simulink model "MAS23_sim"  (R2018b)
settings: Solver=VariableStepAuto  StartTime=0.0  StopTime=tps_sim  MaxStep=1e-4  RelTol=1e-3
values from neighbouring files (symbols this model uses):
  alpha = 4e-3    (= 0.004)    [MAS23_init.m]
  C_in = Cn    (= 643)    [MAS23_init.m]
  Cemn = Cn + pm/Wn    (= 647.177013984)    [MAS23_init.m]
  Concordia = sqrt(2/3)*[1 -0.5 -0.5;0 sqrt(3)/2 -sqrt(3)/2;1/sqrt(2) 1/sqrt(2) 1/sqrt(2)]    [MAS23_init.m]
  decider_R = 1    [MAS23_init.m]
  deciderC = 1    [MAS23_init.m]
  deciderC2 = 1    [MAS23_init.m]
  echauffement = 200    [MAS23_init.m]
  f = u(3)*u(2)/u(1)    [FluxCloche.m]    (also in MAS23_init.m = 0.0131717538735)
  Frdn_max = Frdn*sqrt(2)    [MAS23_init.m]
  IConcordia = inv(Concordia)    [MAS23_init.m]
  IFlux = inv(Flux)    [MAS23_init.m]
  J = 1.92    [MAS23_init.m]
  kc = Cn/Wn    (= 2.06601537836)    [MAS23_init.m]
  Kc = 1.6*3*to_c/sigma/Ts/(P*Msr^2/Lr*Imr_refn/Rs)    [MAS23_init.m]
  Kf = 0.02*3/Tr    [MAS23_init.m]
  Kv = 3    [MAS23_init.m]
  Lr = Lrr-Mr    [MAS23_init.m]
  Ls = Lss-Ms    [MAS23_init.m]
  Msr = 3/2*Msri    [MAS23_init.m]
  N_in = Nn    (= 2972)    [MAS23_init.m]
  P = 1    [MAS23_init.m]
  Rr = Rs    [MAS23_init.m]
  Rs = Rp2    [MAS23_init.m]
  sigma = 1-Msr^2/Ls/Lr    [MAS23_init.m]
  tau = 2    [MAS23_init.m]
  to_c = 0.0055    [MAS23_init.m]
  to_f = 1/(-poleF(2))    [MAS23_init.m]
  to_v = J/k    (= 145.766465001)    [MAS23_init.m]
  Tr = Lr/Rr    [MAS23_init.m]
  Wb = 2*pi*freq    (= 314.159265359)    [MAS23_init.m]
settings Model: Creator=Louis  LastModifiedBy=Louis
settings DataIOCC: SaveOutput=off  SignalLogging=off  DSMLogging=off  SaveTime=off  TimeSaveName=T

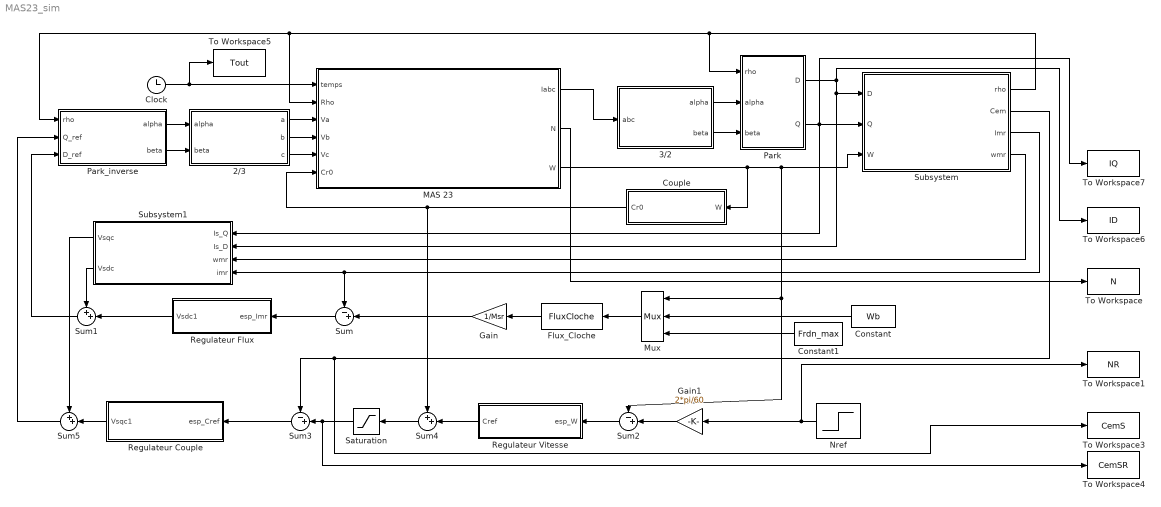
== system MAS23_sim ==
  2/3 : Subsystem
  3/2 : Subsystem
  Clock : Clock
  Constant : Constant  Value=Wb
  Constant1 : Constant  Value=Frdn_max
  Couple : Subsystem
  Flux_Cloche : MATLABFcn  MATLABFcn=FluxCloche  OutputDimensions=1
  Gain : Gain  Gain=1/Msr
  Gain1 : Gain  Gain=2*pi/60
  MAS 23 : Subsystem
      mask Display: image(imread('electricmotor.jpg'));
  Mux : Mux  Inputs=3
  Nref : Step  Time=2  After=N_in  SampleTime=0
  Park : Subsystem
  Park_inverse : Subsystem
  Regulateur Couple : Subsystem
  Regulateur Flux : Subsystem
  Regulateur Vitesse : Subsystem
  Saturation : Saturate  UpperLimit=Cemn  LowerLimit=-Cemn
  Subsystem : Subsystem
  Subsystem1 : Subsystem
  Sum : Sum  Inputs=-+|
  Sum1 : Sum  Inputs=++|
  Sum2 : Sum  Inputs=-+|
  Sum3 : Sum  Inputs=-+|
  Sum4 : Sum  Inputs=++|
  Sum5 : Sum  Inputs=++|
  To Workspace : ToWorkspace  VariableName=N  SampleTime=-1
  To Workspace1 : ToWorkspace  VariableName=NR  SampleTime=-1
  To Workspace3 : ToWorkspace  VariableName=CemS  SampleTime=-1
  To Workspace4 : ToWorkspace  VariableName=CemSR  SampleTime=-1
  To Workspace5 : ToWorkspace  VariableName=Tout  SampleTime=-1
  To Workspace6 : ToWorkspace  VariableName=ID  SampleTime=-1
  To Workspace7 : ToWorkspace  VariableName=IQ  SampleTime=-1
  wires:
  MAS 23/1(Iabc) -> 3/2/1(abc)
  3/2/1(alpha) -> Park/2(alpha)
  3/2/2(beta) -> Park/3(beta)
  Park_inverse/1(alpha) -> 2/3/1(alpha)
  Park_inverse/2(beta) -> 2/3/2(beta)
  2/3/1(a) -> MAS 23/3(Va)
  2/3/2(b) -> MAS 23/4(Vb)
  2/3/3(c) -> MAS 23/5(Vc)
  Subsystem/1(rho) -> Park/1(rho), MAS 23/2(Rho), Park_inverse/1(rho)
  Park/2(Q) -> Subsystem/2(Q), Subsystem1/1(Is_Q), To Workspace7/1
  MAS 23/3(W) -> Couple/1(W), Sum2/1, Mux/1, Subsystem/3(W)
  Park/1(D) -> Subsystem1/2(Is_D), Subsystem/1(D), To Workspace6/1
  Subsystem/4(wmr) -> Subsystem1/3(wmr)
  Subsystem/3(Imr) -> Sum/1, Subsystem1/4(imr)
  Constant/1 -> Mux/2
  Constant1/1 -> Mux/3
  Mux/1 -> Flux_Cloche/1
  Flux_Cloche/1 -> Gain/1
  Gain/1 -> Sum/2
  Sum/1 -> Regulateur Flux/1(esp_Imr)
  Regulateur Flux/1(Vsdc1) -> Sum1/2
  Subsystem1/2(Vsdc) -> Sum1/1
  Sum1/1 -> Park_inverse/3(D_ref)
  Nref/1 -> To Workspace1/1, Gain1/1
  Gain1/1 -> Sum2/2
  Sum2/1 -> Regulateur Vitesse/1(esp_W)
  Subsystem/2(Cem) -> To Workspace3/1, Sum3/1
  Sum3/1 -> Regulateur Couple/1(esp_Cref)
  Regulateur Vitesse/1(Cref) -> Sum4/2
  Saturation/1 -> To Workspace4/1, Sum3/2
  Subsystem1/1(Vsqc) -> Sum5/1
  Sum5/1 -> Park_inverse/2(Q_ref)
  MAS 23/2(N) -> To Workspace/1
  Couple/1(Cr0) -> Sum4/1, MAS 23/6(Cr0)
  Regulateur Couple/1(Vsqc1) -> Sum5/2
  Sum4/1 -> Saturation/1
  Clock/1 -> To Workspace5/1, MAS 23/1(temps)

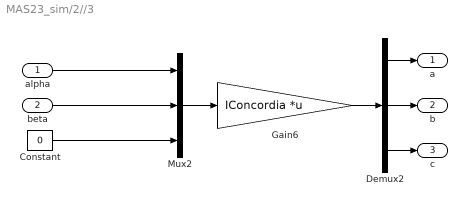
== system MAS23_sim/2//3 ==
  alpha : Inport
  beta : Inport  Port=2
  Constant : Constant  Value=0
  Demux2 : Demux  Outputs=3
  Gain6 : Gain  Gain=IConcordia  Multiplication=Matrix(K*u) (u vector)
  Mux2 : Mux  Inputs=3
  a : Outport
  b : Outport  Port=2
  c : Outport  Port=3
  wires:
  Demux2/1 -> a/1
  Demux2/2 -> b/1
  alpha/1 -> Mux2/1
  Constant/1 -> Mux2/3
  beta/1 -> Mux2/2
  Gain6/1 -> Demux2/1
  Demux2/3 -> c/1
  Mux2/1 -> Gain6/1

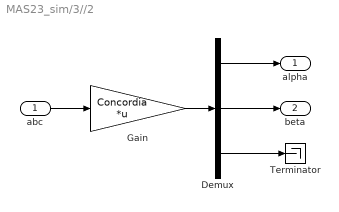
== system MAS23_sim/3//2 ==
  abc : Inport
  Demux : Demux  Outputs=3
  Gain : Gain  Gain=Concordia  Multiplication=Matrix(K*u) (u vector)
  Terminator : Terminator
  alpha : Outport
  beta : Outport  Port=2
  wires:
  Gain/1 -> Demux/1
  Demux/3 -> Terminator/1
  Demux/2 -> beta/1
  abc/1 -> Gain/1
  Demux/1 -> alpha/1

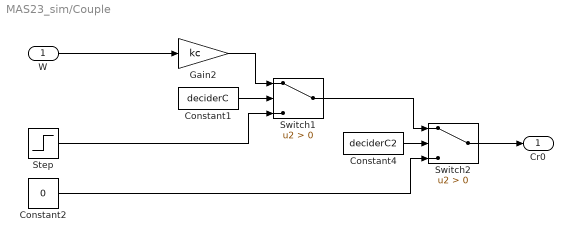
== system MAS23_sim/Couple ==
  W : Inport
  Constant1 : Constant  Value=deciderC
  Constant2 : Constant  Value=0
  Constant4 : Constant  Value=deciderC2
  Gain2 : Gain  Gain=kc
  Step : Step  Time=6  After=C_in  SampleTime=0
  Switch1 : Switch  Criteria=u2 > Threshold
  Switch2 : Switch  Criteria=u2 > Threshold
  Cr0 : Outport
  wires:
  W/1 -> Gain2/1
  Gain2/1 -> Switch1/1
  Constant1/1 -> Switch1/2
  Step/1 -> Switch1/3
  Switch1/1 -> Switch2/1
  Constant2/1 -> Switch2/3
  Constant4/1 -> Switch2/2
  Switch2/1 -> Cr0/1

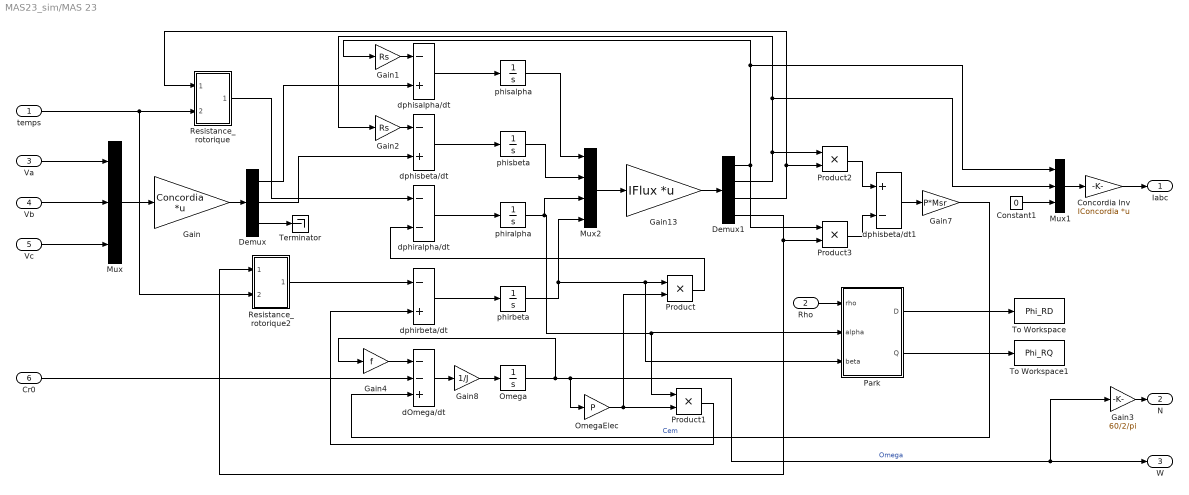
== system MAS23_sim/MAS 23 ==
  temps : Inport
  Rho : Inport  Port=2
  Va : Inport  Port=3
  Vb : Inport  Port=4
  Vc : Inport  Port=5
  Cr0 : Inport  Port=6
  Concordia Inv : Gain  Gain=IConcordia  Multiplication=Matrix(K*u) (u vector)
  Constant1 : Constant  Value=0
  Demux : Demux  Outputs=3
  Demux1 : Demux
  Gain : Gain  Gain=Concordia  Multiplication=Matrix(K*u) (u vector)
  Gain1 : Gain  Gain=Rs
  Gain13 : Gain  Gain=IFlux  Multiplication=Matrix(K*u) (u vector)
  Gain2 : Gain  Gain=Rs
  Gain3 : Gain  Gain=60/2/pi
  Gain4 : Gain  Gain=f
  Gain7 : Gain  Gain=P*Msr
  Gain8 : Gain  Gain=1/J
  Mux : Mux  Inputs=3
  Mux1 : Mux  Inputs=3
  Mux2 : Mux
  Omega : Integrator
  OmegaElec : Gain  Gain=P
  Park : Subsystem
  Product{,1..3} (4 alike) : Product
  Resistance_rotorique : Subsystem
  Resistance_rotorique2 : Subsystem
  Terminator : Terminator
  To Workspace : ToWorkspace  VariableName=Phi_RD  SampleTime=-1
  To Workspace1 : ToWorkspace  VariableName=Phi_RQ  SampleTime=-1
  dOmega/dt : Sum  Inputs=--+
  dphiralpha/dt : Sum  Inputs=--
  dphirbeta/dt : Sum  Inputs=-+
  dphisalpha/dt : Sum  Inputs=-+
  dphisbeta/dt : Sum  Inputs=-+
  dphisbeta/dt1 : Sum  Inputs=+-
  phiralpha : Integrator
  phirbeta : Integrator
  phisalpha : Integrator
  phisbeta : Integrator
  Iabc : Outport
  N : Outport  Port=2
  W : Outport  Port=3
  wires:
  Vc/1 -> Mux/3
  phisalpha/1 -> Mux2/1
  Mux2/1 -> Gain13/1
  Va/1 -> Mux/1
  phirbeta/1 -> Mux2/4, Product/1, Park/3(beta)
  dphisalpha/dt/1 -> phisalpha/1
  Gain13/1 -> Demux1/1
  dphirbeta/dt/1 -> phirbeta/1
  Product/1 -> dphiralpha/dt/2
  Demux/2 -> dphisbeta/dt/2
  Gain/1 -> Demux/1
  Product1/1 -> dphirbeta/dt/2
  phisbeta/1 -> Mux2/2
  Gain7/1 -> dOmega/dt/3  "Cem"
  dphisbeta/dt1/1 -> Gain7/1
  Mux1/1 -> Concordia Inv/1
  Product3/1 -> dphisbeta/dt1/2
  Gain1/1 -> dphisalpha/dt/1
  phiralpha/1 -> Product1/1, Park/2(alpha), Mux2/3
  Demux/3 -> Terminator/1
  Gain2/1 -> dphisbeta/dt/1
  dphisbeta/dt/1 -> phisbeta/1
  Demux/1 -> dphisalpha/dt/2
  Gain8/1 -> Omega/1
  Gain4/1 -> dOmega/dt/1
  Demux1/1 -> Gain1/1, Mux1/1, Product3/1
  Mux/1 -> Gain/1
  Product2/1 -> dphisbeta/dt1/1
  Constant1/1 -> Mux1/3
  Demux1/4 -> Resistance_rotorique2/1(In1), Product3/2
  OmegaElec/1 -> Product1/2, Product/2
  dphiralpha/dt/1 -> phiralpha/1
  Vb/1 -> Mux/2
  Demux1/2 -> Gain2/1, Mux1/2, Product2/1
  dOmega/dt/1 -> Gain8/1
  Omega/1 -> Gain4/1, Gain3/1, W/1, OmegaElec/1  "Omega"
  Demux1/3 -> Resistance_rotorique/1(In1), Product2/2
  Resistance_rotorique2/1(Out1) -> dphirbeta/dt/1
  Resistance_rotorique/1(Out1) -> dphiralpha/dt/1
  Cr0/1 -> dOmega/dt/2
  Concordia Inv/1 -> Iabc/1
  Rho/1 -> Park/1(rho)
  Park/1(D) -> To Workspace/1
  Park/2(Q) -> To Workspace1/1
  temps/1 -> Resistance_rotorique2/2(Time), Resistance_rotorique/2(Time)
  Gain3/1 -> N/1

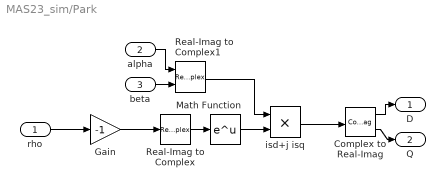
== system MAS23_sim/Park ==
  rho : Inport
  alpha : Inport  Port=2
  beta : Inport  Port=3
  Complex to Real-Imag : ComplexToRealImag
  Gain : Gain  Gain=-1
  Math Function : Math  SaturateOnIntegerOverflow=on
  Real-Imag to Complex : RealImagToComplex  Input=Imag
  Real-Imag to Complex1 : RealImagToComplex
  isd+j isq : Product
  D : Outport
  Q : Outport  Port=2
  wires:
  Complex to Real-Imag/1 -> D/1
  Complex to Real-Imag/2 -> Q/1
  rho/1 -> Gain/1
  alpha/1 -> Real-Imag to Complex1/1
  beta/1 -> Real-Imag to Complex1/2
  Real-Imag to Complex/1 -> Math Function/1
  Real-Imag to Complex1/1 -> isd+j isq/1
  Gain/1 -> Real-Imag to Complex/1
  isd+j isq/1 -> Complex to Real-Imag/1
  Math Function/1 -> isd+j isq/2

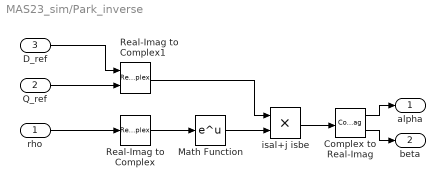
== system MAS23_sim/Park_inverse ==
  rho : Inport
  Q_ref : Inport  Port=2
  D_ref : Inport  Port=3
  Complex to Real-Imag : ComplexToRealImag
  Math Function : Math  SaturateOnIntegerOverflow=on
  Real-Imag to Complex : RealImagToComplex  Input=Imag
  Real-Imag to Complex1 : RealImagToComplex
  isal+j isbe : Product
  alpha : Outport
  beta : Outport  Port=2
  wires:
  Q_ref/1 -> Real-Imag to Complex1/2
  D_ref/1 -> Real-Imag to Complex1/1
  Math Function/1 -> isal+j isbe/2
  isal+j isbe/1 -> Complex to Real-Imag/1
  rho/1 -> Real-Imag to Complex/1
  Real-Imag to Complex1/1 -> isal+j isbe/1
  Real-Imag to Complex/1 -> Math Function/1
  Complex to Real-Imag/2 -> beta/1
  Complex to Real-Imag/1 -> alpha/1

== system MAS23_sim/Regulateur Couple ==
  esp_Cref : Inport
  Cc : TransferFcn  Numerator=[to_c 1]  Denominator=[to_c 0]
  Gain3 : Gain  Gain=Kc
  Vsqc1 : Outport
  wires:
  Gain3/1 -> Cc/1
  esp_Cref/1 -> Gain3/1
  Cc/1 -> Vsqc1/1

== system MAS23_sim/Regulateur Flux ==
  esp_Imr : Inport
  Cp : TransferFcn  Numerator=[to_f 1]  Denominator=[to_f 0]
  Gain1 : Gain  Gain=Kf
  Vsdc1 : Outport
  wires:
  Gain1/1 -> Cp/1
  Cp/1 -> Vsdc1/1
  esp_Imr/1 -> Gain1/1

== system MAS23_sim/Regulateur Vitesse ==
  esp_W : Inport
  Gain4 : Gain  Gain=Kv
  Transfer Fcn : TransferFcn  Numerator=[to_v 1]  Denominator=[to_v 0]
  Cref : Outport
  wires:
  Gain4/1 -> Transfer Fcn/1
  esp_W/1 -> Gain4/1
  Transfer Fcn/1 -> Cref/1

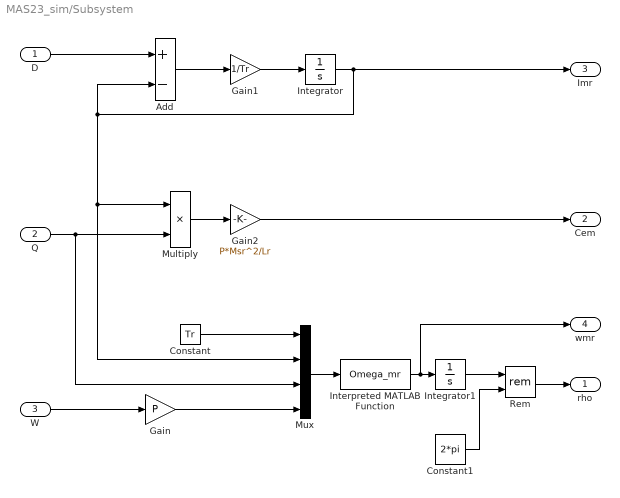
== system MAS23_sim/Subsystem ==
  D : Inport
  Q : Inport  Port=2
  W : Inport  Port=3
  Add : Sum  Inputs=+-
  Constant : Constant  Value=Tr
  Constant1 : Constant  Value=2*pi
  Gain : Gain  Gain=P
  Gain1 : Gain  Gain=1/Tr
  Gain2 : Gain  Gain=P*Msr^2/Lr
  Integrator : Integrator
  Integrator1 : Integrator
  Interpreted MATLAB Function : MATLABFcn  MATLABFcn=Omega_mr  OutputDimensions=1
  Multiply : Product
  Mux : Mux
  Rem : Math  Operator=rem  SaturateOnIntegerOverflow=on
  rho : Outport
  Cem : Outport  Port=2
  Imr : Outport  Port=3
  wmr : Outport  Port=4
  wires:
  W/1 -> Gain/1
  D/1 -> Add/1
  Integrator/1 -> Imr/1, Multiply/1, Mux/2, Add/2
  Add/1 -> Gain1/1
  Gain1/1 -> Integrator/1
  Q/1 -> Multiply/2, Mux/3
  Multiply/1 -> Gain2/1
  Gain2/1 -> Cem/1
  Integrator1/1 -> Rem/1
  Constant1/1 -> Rem/2
  Gain/1 -> Mux/4
  Constant/1 -> Mux/1
  Interpreted MATLAB Function/1 -> wmr/1, Integrator1/1
  Mux/1 -> Interpreted MATLAB Function/1
  Rem/1 -> rho/1

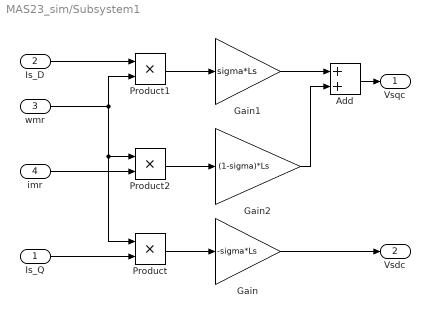
== system MAS23_sim/Subsystem1 ==
  Is_Q : Inport
  Is_D : Inport  Port=2
  wmr : Inport  Port=3
  imr : Inport  Port=4
  Add : Sum
  Gain : Gain  Gain=-sigma*Ls
  Gain1 : Gain  Gain=sigma*Ls
  Gain2 : Gain  Gain=(1-sigma)*Ls
  Product : Product
  Product1 : Product
  Product2 : Product
  Vsqc : Outport
  Vsdc : Outport  Port=2
  wires:
  imr/1 -> Product2/2
  Is_Q/1 -> Product/2
  wmr/1 -> Product1/2, Product/1, Product2/1
  Is_D/1 -> Product1/1
  Add/1 -> Vsqc/1
  Product1/1 -> Gain1/1
  Gain/1 -> Vsdc/1
  Gain2/1 -> Add/2
  Product/1 -> Gain/1
  Gain1/1 -> Add/1
  Product2/1 -> Gain2/1

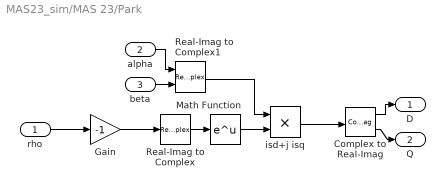
== system MAS23_sim/MAS 23/Park ==
  rho : Inport
  alpha : Inport  Port=2
  beta : Inport  Port=3
  Complex to Real-Imag : ComplexToRealImag
  Gain : Gain  Gain=-1
  Math Function : Math  SaturateOnIntegerOverflow=on
  Real-Imag to Complex : RealImagToComplex  Input=Imag
  Real-Imag to Complex1 : RealImagToComplex
  isd+j isq : Product
  D : Outport
  Q : Outport  Port=2
  wires:
  Complex to Real-Imag/1 -> D/1
  Complex to Real-Imag/2 -> Q/1
  rho/1 -> Gain/1
  alpha/1 -> Real-Imag to Complex1/1
  beta/1 -> Real-Imag to Complex1/2
  Real-Imag to Complex/1 -> Math Function/1
  Real-Imag to Complex1/1 -> isd+j isq/1
  Gain/1 -> Real-Imag to Complex/1
  isd+j isq/1 -> Complex to Real-Imag/1
  Math Function/1 -> isd+j isq/2

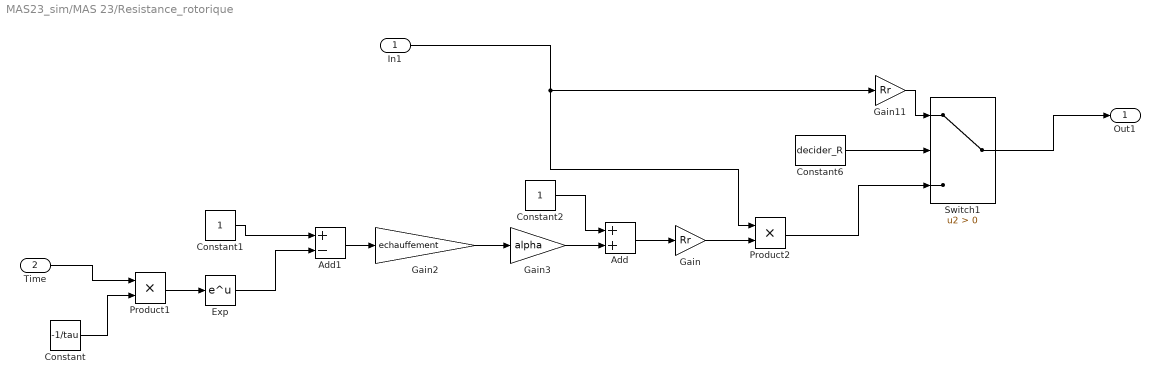
== system MAS23_sim/MAS 23/Resistance_rotorique ==
  In1 : Inport
  Time : Inport  Port=2
  Add : Sum
  Add1 : Sum  Inputs=+-
  Constant : Constant  Value=-1/tau
  Constant1 : Constant
  Constant2 : Constant
  Constant6 : Constant  Value=decider_R
  Exp : Math  SaturateOnIntegerOverflow=on
  Gain : Gain  Gain=Rr
  Gain11 : Gain  Gain=Rr
  Gain2 : Gain  Gain=echauffement
  Gain3 : Gain  Gain=alpha
  Product1 : Product
  Product2 : Product
  Switch1 : Switch  Criteria=u2 > Threshold
  Out1 : Outport
  wires:
  Product2/1 -> Switch1/3
  Gain/1 -> Product2/2
  Add/1 -> Gain/1
  Constant2/1 -> Add/1
  Gain3/1 -> Add/2
  Gain2/1 -> Gain3/1
  Add1/1 -> Gain2/1
  Constant1/1 -> Add1/1
  Exp/1 -> Add1/2
  Constant/1 -> Product1/2
  Product1/1 -> Exp/1
  Time/1 -> Product1/1
  In1/1 -> Product2/1, Gain11/1
  Switch1/1 -> Out1/1
  Constant6/1 -> Switch1/2
  Gain11/1 -> Switch1/1

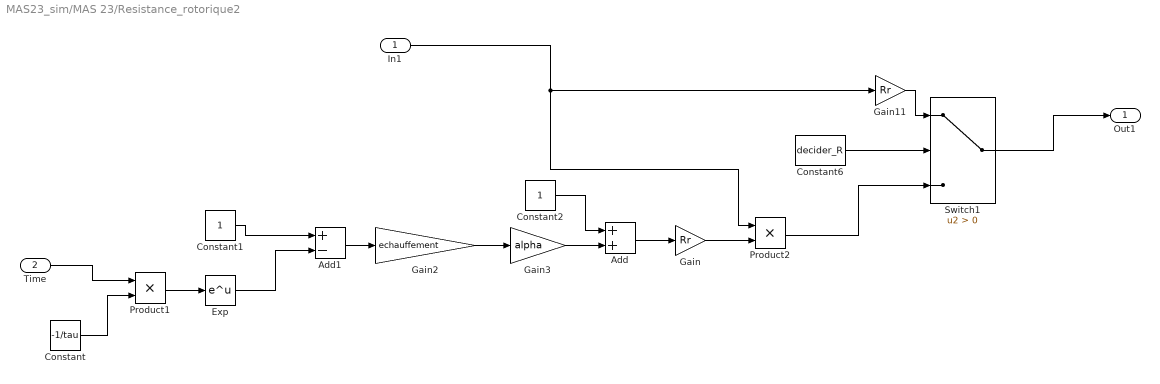
== system MAS23_sim/MAS 23/Resistance_rotorique2 ==
  In1 : Inport
  Time : Inport  Port=2
  Add : Sum
  Add1 : Sum  Inputs=+-
  Constant : Constant  Value=-1/tau
  Constant1 : Constant
  Constant2 : Constant
  Constant6 : Constant  Value=decider_R
  Exp : Math  SaturateOnIntegerOverflow=on
  Gain : Gain  Gain=Rr
  Gain11 : Gain  Gain=Rr
  Gain2 : Gain  Gain=echauffement
  Gain3 : Gain  Gain=alpha
  Product1 : Product
  Product2 : Product
  Switch1 : Switch  Criteria=u2 > Threshold
  Out1 : Outport
  wires:
  Gain11/1 -> Switch1/1
  Constant6/1 -> Switch1/2
  Switch1/1 -> Out1/1
  In1/1 -> Gain11/1, Product2/1
  Time/1 -> Product1/1
  Product1/1 -> Exp/1
  Constant/1 -> Product1/2
  Exp/1 -> Add1/2
  Constant1/1 -> Add1/1
  Add1/1 -> Gain2/1
  Gain2/1 -> Gain3/1
  Gain3/1 -> Add/2
  Constant2/1 -> Add/1
  Add/1 -> Gain/1
  Gain/1 -> Product2/2
  Product2/1 -> Switch1/3
